simulink model "BoostConverter"  (R2023b)
settings: Solver=VariableStepAuto  StartTime=0.0  StopTime=0.308  MaxStep=1e-4  RelTol=1e-4  EnableMultiTasking=on
libraries: spsSeriesRLCBranchLib x3, spsCurrentMeasurementLib x1, spsDiodeLib x1, spsMosfetLib x1, spsPWMGeneratorDCDCLib x1, spsDCVoltageSourceLib x1, spsVoltageMeasurementLib x1, spspowerguiLib x1
settings Model: Creator=The MathWorks, Inc.  LastModifiedBy=Admin
settings SolverCC: AlgebraicLoopSolver=TrustRegion  SolverResetMethod=Robust
settings OptimizationCC: EfficientFloat2IntCast=on  LifeSpan=inf
settings DebuggingCC: ReadBeforeWriteMsg=DisableAll  WriteAfterWriteMsg=DisableAll  WriteAfterReadMsg=DisableAll  UnconnectedInputMsg=warning  UnconnectedOutputMsg=warning  UnconnectedLineMsg=warning  UniqueDataStoreMsg=error  StrictBusMsg=ErrorOnBusTreatedAsVector  SFUnexpectedBacktrackingDiag=warning  SFNoUnconditionalDefaultTransitionDiag=warning  SFExecutionAtInitializationDiag=none  ArithmeticOperatorsInVariantConditions=warning
settings ModelReferenceCC: UpdateModelReferenceTargets=IfOutOfDate  EnableRefExpFcnMdlSchedulingChecks=on
settings SFSimCC: SFSimEcho=off  SimUseLocalCustomCode=off  CustomCodeUndefinedFunction=UseInterfaceOnly
settings RTWCC: RTWUseLocalCustomCode=off
settings CodeAppCC: StateflowObjectComments=on
settings GRTTargetCC: TargetLangStandard=C89/C90 (ANSI)
settings ConfigComp: CovMetricSettings=dw  CovSaveCumulativeToWorkspaceVar=on  CovSaveSingleToWorkspaceVar=on  CovExternalEMLEnable=off
settings SimscapeCC: SimscapeNormalizeSystem=off  SimscapeNominalValues={1, 'bar'; 1, 'cm^3/s'; 1, 'bar*kg/s'; 1, 'kJ/kg'; 1, 'kW'; }

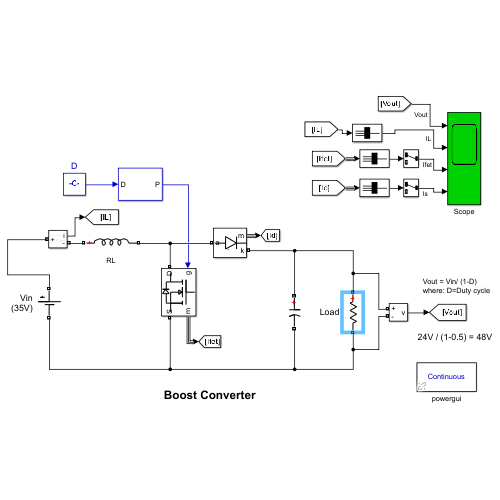
[thumbnail: Simulink's stored preview of the top-level diagram]
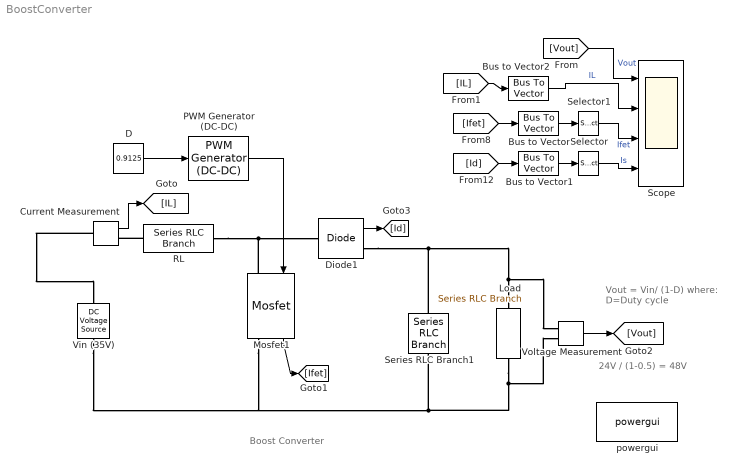
== system BoostConverter ==
  note: 24V / (1-0.5) = 48V
  note: Vout = Vin/ (1-D)
      | where: D=Duty cycle
  note: Boost Converter
  Bus to Vector : BusToVector
  Bus to Vector1 : BusToVector
  Bus to Vector2 : BusToVector
  Current Measurement : spsCurrentMeasurementLib/Current Measurement  PhasorSimulation=off  OutputType=Complex  PSBequivalent=0
  D : Constant  Value=0.9125
  Diode1 : spsDiodeLib/Diode  Ron=0  Lon=0  Vf=0  IC=0  UseSnubber=off  Rs=inf  Cs=inf  Measurements=on
  Load : spsSeriesRLCBranchLib/Series RLC Branch  LConnTagsString=__new0  RConnTagsString=__new0  BranchType=R  Resistance=160  Inductance=200e-6  SetiL0=off  InitialCurrent=0  Capacitance=400e-6  Setx0=off  InitialVoltage=0  Measurements=None
  Mosfet1 : spsMosfetLib/Mosfet  Ron=0  Lon=0  Rd=0  Vfd=0  IC=0  Rs=inf  Cs=inf  Measurements=on
  PWM Generator (DC-DC) : spsPWMGeneratorDCDCLib/PWM Generator (DC-DC)  Fsw=20e3  Ts=0
  RL : spsSeriesRLCBranchLib/Series RLC Branch  LConnTagsString=__new0  RConnTagsString=__new0  BranchType=L  Resistance=0  Inductance=55.89e-6  SetiL0=off  InitialCurrent=0  Capacitance=1e-6  Setx0=off  InitialVoltage=0  Measurements=None
  Scope : Scope  NumInputPorts=4
  Selector : Selector  InputPortWidth=2  IndexOptions=Index vector (dialog)  Indices=1  OutputSizes=1
  Selector1 : Selector  InputPortWidth=2  IndexOptions=Index vector (dialog)  Indices=1  OutputSizes=1
  Series RLC Branch1 : spsSeriesRLCBranchLib/Series RLC Branch  LConnTagsString=__new0  RConnTagsString=__new0  BranchType=C  Resistance=1e-4  Inductance=200e-6  SetiL0=off  InitialCurrent=0  Capacitance=2.85e-6  Setx0=off  InitialVoltage=40  Measurements=None
  Vin (35V) : spsDCVoltageSourceLib/DC Voltage Source  Amplitude=35  Measurements=None
  Voltage Measurement : spsVoltageMeasurementLib/Voltage Measurement  PhasorSimulation=off  OutputType=Complex  PSBequivalent=0
  powergui : spspowerguiLib/powergui  Priority=1  SimulationMode=Continuous  SampleTime=50e-6  frequency=60  Iterations=50  frequencyindice=0  Pbase=100e6  ErrMax=1e-4  UnitsV=kV  UnitsW=MW  buscounter=0  FunctionMessages=off  echomessages=off  EnableUseOfTLC=off  CurrentSourceSwitches=off  DisableSnubberDevices=off  DisableRonSwitches=off  DisableVfSwitches=off  DisplayEquations=off  AutomaticDiscreteSolvers=off  SolverType=Tustin/Backward Euler (TBE)  Interpol=off  ExternalGateDelay=off  methode=off  Ts=100  x0status=blocks  SPID=on  SwTol=0  HookPort=off  NonlinearTolerance=1e-4  nMaxIteration=100  ContinueOnMaxIteration=off  RestoreLinks=warning  ResistiveCurrentMeasurement=off  Frange=[0:2:500]  Ylog=off  Xlog=on  ShowGrid=off  save=off  variable=ZData  structure=0  ZoomFFT=off  StartTime=0.0  cycles=1  DisplayStyle=1  fundamental=60  FreqAxis=off  MaxFrequency=1000  frequencyindicesteady=1  RmsSteady=1  display=off
  wires:
  Voltage Measurement/1 -> [Vout]
  [Ifet] -> Bus to Vector/1
  [Id] -> Bus to Vector1/1
  Selector1/1 -> Scope/3  "Ifet"
  Selector/1 -> Scope/4  "Is"
  [Vout] -> Scope/1  "Vout"
  Mosfet1/1 -> [Ifet]
  Diode1/1 -> [Id]
  PWM Generator (DC-DC)/1 -> Mosfet1/1
  D/1 -> PWM Generator (DC-DC)/1
  Bus to Vector/1 -> Selector1/1
  Bus to Vector1/1 -> Selector/1
  Current Measurement/1 -> [IL]
  Bus to Vector2/1 -> Scope/2  "IL"
  [IL] -> Bus to Vector2/1
  connections:
  Load/RConn1 -- Vin (35V)/LConn1 -- Mosfet1/RConn1 -- Series RLC Branch1/RConn1 -- Voltage Measurement/LConn2
  Series RLC Branch1/LConn1 -- Diode1/RConn1 -- Voltage Measurement/LConn1 -- Load/LConn1
  RL/LConn1 -- Current Measurement/RConn1
  RL/RConn1 -- Mosfet1/LConn1 -- Diode1/LConn1
  Current Measurement/LConn1 -- Vin (35V)/RConn1
